simulink model "Powertrain_Simulation"  (R2017b)
settings: Solver=FixedStepAuto  StartTime=0.0  StopTime=Inf  MinStep=0.01  RelTol=1e-3
values from neighbouring files (symbols this model uses):
  Rear_Sprocket_FirstGear = Rear_Sprocket    [Optimize_SingleSpeedGearRatio.m]
  Rear_Sprocket_SecondGear = Rear_Sprocket    [Optimize_SingleSpeedGearRatio.m]
undefined symbols (not defined in the file or in its folder): A1, AIR, C1, C2, COOLANT, cp, Elevation_Profile, EM, flowrate, hA1, k12, M, M2, MOT, RAD, Velocity_Profile
libraries: simulink x5
(part 1 of 2)
settings Model: Creator=salyer.103  LastModifiedBy=ra067402
settings SolverCC: ZeroCrossAlgorithm=Adaptive
settings CodeAppCC: StateflowObjectComments=on

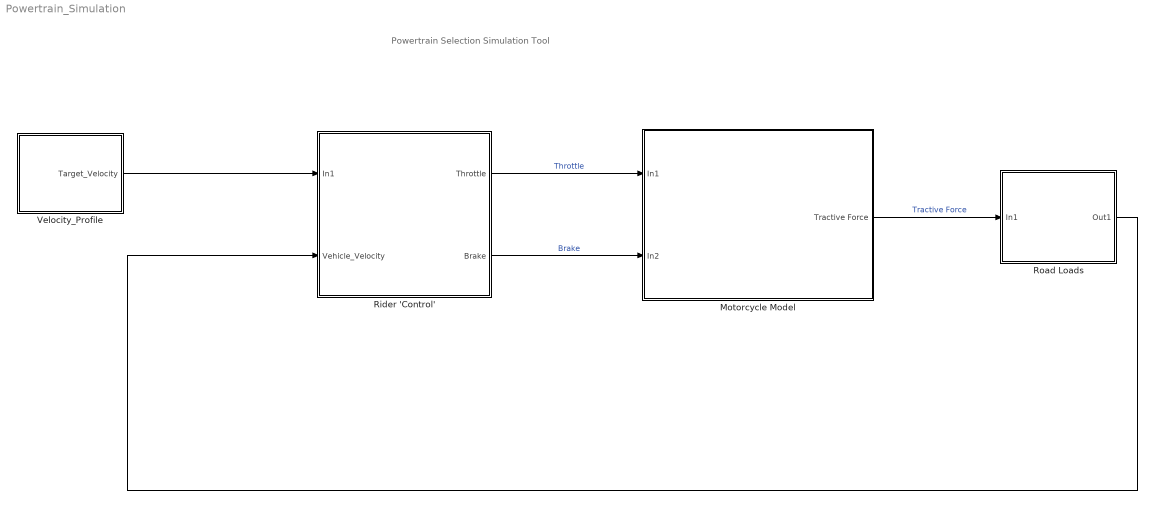
== system Powertrain_Simulation ==
  note: Powertrain Selection Simulation Tool
  Motorcycle Model : Subsystem  mask{Wheel_Radius=0.3, Final_Drive_Eff=0.92, Max_Brake_Torque=4000, Total_Mass=330, EM_MC_Selection=Ideal_TomegaCurve, b=0.728, h=0.72, g=9.81, p=1.4, mu_r=1, Front_Sprocket=21, Regen_Percent=100}
      mask prompts: Wheel_Radius "Wheel Radius (m)"; Final_Drive_Eff "Efficiency of Drivetrain"; Max_Brake_Torque "Maximum Braking Torque (Nm)"; Total_Mass "Vehicle Total Mass (kg)"; EM_MC_Selection "Motor-MC Combo"; b "Distance from Rear Wheel to CG (m)"; h "Height of CG from ground (m)"; g "Gravity (m/s2)"; p "Wheelbase (m)"; mu_r "Rear Wheel Coefficient of Friction"; Front_Sprocket "Front Sprocket Teeth"; Regen_Percent "Percentage of Max Regen (%)"
      mask init:
      | Initialize_Powertrain
      mask TypeOptions EM_MC_Selection: emrax268_pm150dz | RemyHVH25090s | Ideal_TomegaCurve
      mask Display: image('\\home2.coeit.osu.edu\s\salyer.103\Documents\GrabCAD\RW-4\Layout Space\Zach Salyer\Powertrain Simulation\Mask Pictures\bike.JPG');
  Rider 'Control' : Subsystem  mask{kp=5, ki=0, kd=0}
      mask Display: image('\\home2.coeit.osu.edu\s\salyer.103\Documents\GrabCAD\RW-4\Layout Space\Zach Salyer\Powertrain Simulation\Mask Pictures\helmet.jpg');
  Road Loads : Subsystem  mask{rowA=1, Wind_Speed=0, Cda=0.38, ElevationProfile=IOM_Elevation_Profile}
      mask prompts: rowA "Air Density"; Wind_Speed "Wind Speed (m/s)"; Cda "Cd * Frontal Area"; ElevationProfile "Course Elevation Profile"
      mask init:
      | Initialize_Elevation
      mask TypeOptions ElevationProfile: IOM_Elevation_Profile
  Velocity_Profile : Subsystem  mask{Circuit_Selection=IOM}
      mask prompts: Circuit_Selection "Circuit"
      mask init:
      | Initialize_Circuit
      mask TypeOptions Circuit_Selection: IOM
      mask Display: image('\\home2.coeit.osu.edu\s\salyer.103\Documents\GrabCAD\RW-4\Layout Space\Zach Salyer\Powertrain Simulation\Mask Pictures\VelocityProfile.png');
  wires:
  Velocity_Profile/1(Target_Velocity) -> Rider 'Control'/1(In1)
  Rider 'Control'/1(Throttle) -> Motorcycle Model/1(In1)  "Throttle"
  Rider 'Control'/2(Brake) -> Motorcycle Model/2(In2)  "Brake"
  Motorcycle Model/1(Tractive Force) -> Road Loads/1(In1)  "Tractive Force"
  Road Loads/1(Out1) -> Rider 'Control'/2(Vehicle_Velocity)

== system Powertrain_Simulation/Motorcycle Model ==
  note: When Rear Braking Strategy is added, will need to move pack energy req block
      | B/c negative torque applied gives regen to pack
      |
      | To determine actual applied torque prior to the wheel block we will  need to modulate torque based on
      | wheel slip from the rider model
  In1 : Inport
  In2 : Inport  Port=2
  Braking/Throttle Strategy : Subsystem
  Front Brakes : Subsystem
      mask Display: image('\\home2.coeit.osu.edu\s\salyer.103\Documents\GrabCAD\RW-4\Layout Space\Zach Salyer\Powertrain Simulation\Mask Pictures\motoBrake.JPG');
  Front Wheel (Limits Tractive Force) : Subsystem
      mask Display: image('\\home2.coeit.osu.edu\s\salyer.103\Documents\GrabCAD\RW-4\Layout Space\Zach Salyer\Powertrain Simulation\Mask Pictures\frTire_pirelli.JPG');
  Pack Energy Req : Subsystem
      mask Display: image('\\home2.coeit.osu.edu\s\salyer.103\Documents\GrabCAD\RW-4\Layout Space\Zach Salyer\Powertrain Simulation\Mask Pictures\pack.JPG');
  Powertrain : Subsystem
      mask Display: image('\\home2.coeit.osu.edu\s\salyer.103\Documents\GrabCAD\RW-4\Layout Space\Zach Salyer\Powertrain Simulation\Mask Pictures\bike_powertrain.JPG');
  Rear Brakes : Subsystem
      mask Display: image('\\home2.coeit.osu.edu\s\salyer.103\Documents\GrabCAD\RW-4\Layout Space\Zach Salyer\Powertrain Simulation\Mask Pictures\motoBrake.JPG');
  Rear Wheel (Limits Tractive Force) : Subsystem
      mask Display: image('\\home2.coeit.osu.edu\s\salyer.103\Documents\GrabCAD\RW-4\Layout Space\Zach Salyer\Powertrain Simulation\Mask Pictures\rrTire_pirelli.JPG');
  Sum : Sum  Inputs=+|+
  Sum1 : Sum  Inputs=++|
  To Workspace : ToWorkspace  VariableName=RearWhlForce  SampleTime=-1
  To Workspace1 : ToWorkspace  VariableName=FrontWhlForce  SaveFormat=Timeseries  SampleTime=-1
  Transmission : Subsystem
      mask Display: image('\\home2.coeit.osu.edu\s\salyer.103\Documents\GrabCAD\RW-4\Layout Space\Zach Salyer\Powertrain Simulation\Mask Pictures\gear.jpg');
  Vehicle Parameters : Subsystem
  Tractive Force : Outport
  wires:
  Sum/1 -> Tractive Force/1  "Tractive Force"
  Powertrain/1(Motor Torque) -> Transmission/1(Motor Torque)
  Front Brakes/1(Front Wheel Torque) -> Front Wheel (Limits Tractive Force)/1(In1)
  Front Wheel (Limits Tractive Force)/1(Out2) -> To Workspace1/1, Sum/2
  Rear Wheel (Limits Tractive Force)/1(Out1) -> To Workspace/1, Sum/1, Pack Energy Req/1(In1)
  In1/1 -> Braking/Throttle Strategy/1(In1)  "Throttle"
  Braking/Throttle Strategy/2(Out2) -> Powertrain/1(Throttle)
  In2/1 -> Braking/Throttle Strategy/2(In2)  "Brake"
  Braking/Throttle Strategy/3(Out3) -> Front Brakes/1(Throttle)
  Transmission/1(Out1) -> Sum1/2  "Motor Torque"
  Rear Brakes/1(Front Wheel Torque) -> Sum1/1  "Rear Brake Torque"
  Sum1/1 -> Rear Wheel (Limits Tractive Force)/1(In1)  "Total Torque"
  Braking/Throttle Strategy/1(Out1) -> Rear Brakes/1(Throttle)

== system Powertrain_Simulation/Rider 'Control' ==
  note: Note: This literally just does full throttle is speed < target speed and full brake if speed > target speed
      |
      | It also has a very small derivative gain to keep the simulation from getting stuck if speed = target speed
  note: If positive, accelerate
      | If negative, brake
  note: Tune PID Controller Later/Make Improved Rider Model
  In1 : Inport
  Vehicle_Velocity : Inport  Port=2
  " " : Gain  Gain=ki
  "  " : Gain  Gain=kp
  "   " : Gain  Gain=kd
  Brake Limit : Saturate  UpperLimit=0  LowerLimit=-1  ZeroCross=off
  Derivative : Derivative
  Integrator : Integrator
  Make Brake 0 or 1 : Rounding
  Make Throttle 0 or 1 : Rounding  Operator=ceil
  Scope : Scope
  Sum : Sum  Inputs=+-
  Sum1 : Sum  Inputs=+++
  T : Scope
  Throttle Limit : Saturate  UpperLimit=1  LowerLimit=0  ZeroCross=off
  Throttle : Outport
  Brake : Outport  Port=2
  wires:
  Vehicle_Velocity/1 -> Sum/2  "Velocity"
  In1/1 -> Scope/1, Sum/1  "Target_Velocity"
  "  "/1 -> Sum1/1
  Sum/1 -> "  "/1, " "/1, "   "/1
  Throttle Limit/1 -> Make Throttle 0 or 1/1  "Throttle"
  Make Throttle 0 or 1/1 -> T/1, Throttle/1
  Make Brake 0 or 1/1 -> Brake/1
  " "/1 -> Integrator/1
  Integrator/1 -> Sum1/2
  "   "/1 -> Derivative/1
  Derivative/1 -> Sum1/3
  Sum1/1 -> Brake Limit/1, Throttle Limit/1
  Brake Limit/1 -> Make Brake 0 or 1/1  "Brake"

== system Powertrain_Simulation/Road Loads ==
  In1 : Inport
  Enviornment : Subsystem
  To Workspace : ToWorkspace  VariableName=Vehicle_Velocity  SampleTime=-1
      settings: Save2DSignal=2-D array (concatenate along first dimension)
  To Workspace1 : ToWorkspace  VariableName=resistanceforce  SampleTime=-1
      settings: Save2DSignal=2-D array (concatenate along first dimension)
  Vehicle Loads : Subsystem
  Vehicle_speed_Calculation : Subsystem
  Out1 : Outport
  tag scope: Vehicle_Velocity_ms=global
  wires:
  In1/1 -> Vehicle_speed_Calculation/1(In1)  "Tractive Force"
  Vehicle_speed_Calculation/1(F (N)1) -> To Workspace/1, Out1/1, [Vehicle_Velocity_ms]  "Velocity"
  Vehicle Loads/1(F (N)) -> To Workspace1/1, Vehicle_speed_Calculation/2(In3)

== system Powertrain_Simulation/Velocity_Profile ==
  Constant : Constant  Value=Velocity_Profile.distance(end)
  Relational Operator1 : RelationalOperator  RndMeth=Nearest  InputSameDT=on
  Stop Simulation : Stop
  Vehicle_Target_Speed : Lookup  InputValues=Velocity_Profile.distance  Table=Velocity_Profile.velocity  LookUpMeth=Interpolation-Use End Values  SaturateOnIntegerOverflow=on
  Target_Velocity : Outport
  wires:
  Vehicle_Target_Speed/1 -> Target_Velocity/1  "Target_Velocity"
  Constant/1 -> Relational Operator1/2
  Relational Operator1/1 -> Stop Simulation/1
  [Distance_Total_m] -> Relational Operator1/1, Vehicle_Target_Speed/1

== system Powertrain_Simulation/Motorcycle Model/Braking//Throttle Strategy ==
  note: Notes:
      | -No Rear Brake currently being used, no point in using it until we have a better rider model
      | -If throttle = 0, then switch to -1 to request negative torque
      | -All brake request is front brake
  In1 : Inport
  In2 : Inport  Port=2
  Constant : Constant  Value=0
  Constant1 : Constant  Value=-1
  Gain : Gain
  Switch : Switch  Criteria=u2 > Threshold
  Out1 : Outport
  Out2 : Outport  Port=2
  Out3 : Outport  Port=3
  wires:
  Constant/1 -> Out1/1  "Rear Brake Request"
  In1/1 -> Switch/1, Switch/2  "Throttle Request"
  In2/1 -> Gain/1  "Brake Request"
  Gain/1 -> Out3/1  "Front Brake Request"
  Constant1/1 -> Switch/3
  Switch/1 -> Out2/1  "Torque Request"

== system Powertrain_Simulation/Motorcycle Model/Front Brakes ==
  Throttle : Inport
  Multiply : Product  Inputs=**
  Front Wheel Torque : Outport
  wires:
  Throttle/1 -> Multiply/1  "Brake"
  [Max_Brake_Torque] -> Multiply/2
  Multiply/1 -> Front Wheel Torque/1  "Front Wheel Torque"

== system Powertrain_Simulation/Motorcycle Model/Front Wheel (Limits Tractive Force) ==
  In1 : Inport
  Constant : Constant  Value=0
  Constant1 : Constant  Value=0
  Divide : Product  Inputs=*/
  Dynamic Front Wheel Load * mu : Fcn  Expr=-mu_r*Total_Mass*g*b/p + u(1)*h/p
  Stoppie Limit Brake Force : Constant  Value=-Total_Mass*g*(p-b)/h
  Stoppie Limited Brake Force : simulink/Discontinuities/Saturation Dynamic  OutMin=[]  OutMax=[]  OutDataTypeStr=Inherit: Same as second input  OutDataType=fixdt(1, 16)  OutScaling=2^-10  DoSatur=off
  Sum1 : Sum
  To Workspace : ToWorkspace  VariableName=FrictionLimit  SaveFormat=Timeseries  SampleTime=-1
  Traction Limited Brake Force : simulink/Discontinuities/Saturation Dynamic  OutMin=[]  OutMax=[]  OutDataTypeStr=Inherit: Same as second input  OutDataType=fixdt(1, 16)  OutScaling=2^-10  DoSatur=off
  Out2 : Outport
  tag scope: Front_Brake_Force=global
  wires:
  In1/1 -> Divide/1  "Front Wheel Torque"
  Stoppie Limited Brake Force/1 -> [Front_Brake_Force], Out2/1  "Tractive Force"
  Divide/1 -> Traction Limited Brake Force/2
  [Fr_Wheel_Radius] -> Divide/2
  [Front_Brake_Force] -> Sum1/1
  [Rear_Brake_Force] -> Sum1/2
  Sum1/1 -> Dynamic Front Wheel Load * mu/1
  Dynamic Front Wheel Load * mu/1 -> To Workspace/1, Traction Limited Brake Force/3
  Constant/1 -> Traction Limited Brake Force/1
  Traction Limited Brake Force/1 -> Stoppie Limited Brake Force/2
  Constant1/1 -> Stoppie Limited Brake Force/1
  Stoppie Limit Brake Force/1 -> Stoppie Limited Brake Force/3

== system Powertrain_Simulation/Motorcycle Model/Pack Energy Req ==
  In1 : Inport
  Convert W-s to kW-h : Gain  Gain=1/3600/1000
  Divide : Product  Inputs=*/
  Gain : Gain  Gain=1/1000
  Integrator : Integrator
  Product : Product
  Product1 : Product
  To Workspace : ToWorkspace  VariableName=Motor_Torque_Limited  SampleTime=-1
      settings: Save2DSignal=2-D array (concatenate along first dimension)
  To Workspace1 : ToWorkspace  VariableName=Power  SampleTime=-1
      settings: Save2DSignal=2-D array (concatenate along first dimension)
  To Workspace2 : ToWorkspace  VariableName=Energy_req  SampleTime=-1
      settings: Save2DSignal=2-D array (concatenate along first dimension)
  rpm to rad/s : Gain  Gain=1/60*2*pi
  wires:
  In1/1 -> Product1/1  "Tractive Force"
  Convert W-s to kW-h/1 -> To Workspace2/1
  [EM_RPM] -> rpm to rad/s/1
  Integrator/1 -> Convert W-s to kW-h/1  "Energy"
  rpm to rad/s/1 -> Product/2
  Product/1 -> Gain/1, Integrator/1  "Power (W)"
  Divide/1 -> To Workspace/1, Product/1  "Motor Torque Actual"
  [Rr_Wheel_Radius] -> Product1/2
  Product1/1 -> Divide/1  "Whl Torque"
  [Final_Drive_Ratio] -> Divide/2
  Gain/1 -> To Workspace1/1

== system Powertrain_Simulation/Motorcycle Model/Powertrain ==
  note: Find max torque available based on RPM
  note: Apply max torque (sign will depend on if throttle is positive or negative - regen or accelerate)
      | Apply gain for regen percentage to decrease from max torque is desired
  Throttle : Inport
  Divide : Product  Inputs=**
  EM Max Torque Curve : Lookup  InputValues=EM.N_RPM  Table=EM.T_max_Peak  LookUpMeth=Interpolation-Use End Values  SaturateOnIntegerOverflow=on
  Gain : Gain  Gain=Regen_Percent/100
  Goto : Goto  Commented=on  GotoTag=EM_Torque  TagVisibility=global
  Powertrain Thermal Model : Subsystem  Commented=on
  Switch : Switch  Criteria=u2 > Threshold
  To Workspace : ToWorkspace  VariableName=EM_RPM  SampleTime=-1
      settings: Save2DSignal=2-D array (concatenate along first dimension)
  To Workspace2 : ToWorkspace  VariableName=motorT  SaveFormat=Timeseries  SampleTime=-1
  Motor Torque : Outport
  wires:
  Throttle/1 -> Divide/1  "Throttle"
  Divide/1 -> To Workspace2/1, Goto/1, Switch/2, Gain/1, Switch/1  "Motor Torque"
  [EM_RPM] -> To Workspace/1, EM Max Torque Curve/1  "EM_RPM"
  EM Max Torque Curve/1 -> [T_Max_from_EM]  "Max Torque"
  [T_Max_from_EM] -> Divide/2
  Switch/1 -> Motor Torque/1  "Motor Torque"
  Gain/1 -> Switch/3

== system Powertrain_Simulation/Motorcycle Model/Rear Brakes ==
  Throttle : Inport
  Multiply : Product  Inputs=**
  Front Wheel Torque : Outport
  wires:
  Throttle/1 -> Multiply/1  "Brake"
  [Max_Brake_Torque] -> Multiply/2
  Multiply/1 -> Front Wheel Torque/1  "Rear Wheel Torque"

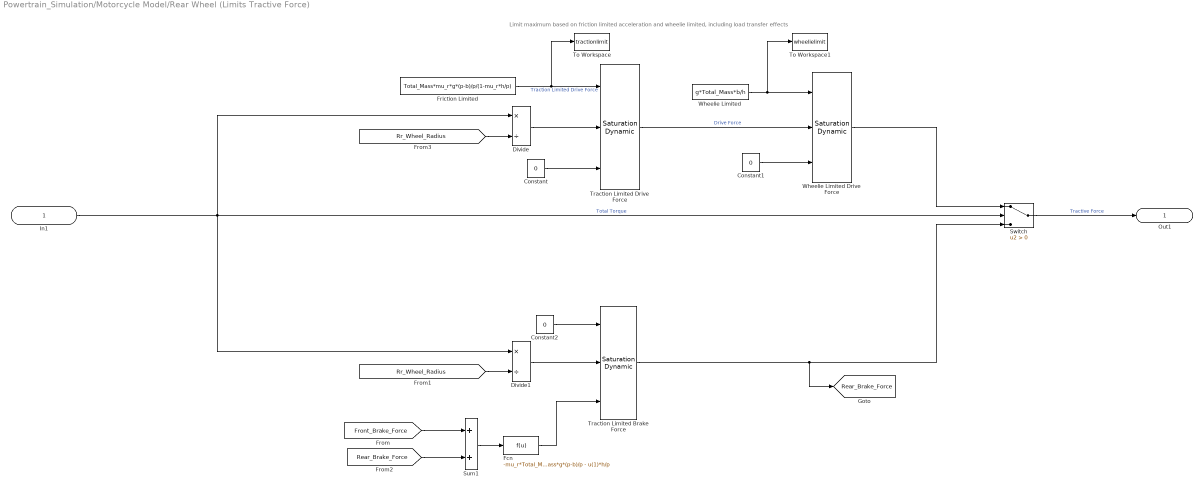
== system Powertrain_Simulation/Motorcycle Model/Rear Wheel (Limits Tractive Force) ==
  note: Limit maximum based on friction limited acceleration and wheelie limited, including load transfer effects
  In1 : Inport
  Constant : Constant  Value=0
  Constant1 : Constant  Value=0
  Constant2 : Constant  Value=0
  Divide : Product  Inputs=*/
  Divide1 : Product  Inputs=*/
  Fcn : Fcn  Expr=-mu_r*Total_Mass*g*(p-b)/p - u(1)*h/p
  Friction Limited : Constant  Value=Total_Mass*mu_r*g*(p-b)/p/(1-mu_r*h/p)
  Sum1 : Sum
  Switch : Switch  Criteria=u2 > Threshold
  To Workspace : ToWorkspace  VariableName=tractionlimit  SaveFormat=Timeseries  SampleTime=-1
  To Workspace1 : ToWorkspace  VariableName=wheelielimit  SaveFormat=Timeseries  SampleTime=-1
  Traction Limited Brake Force : simulink/Discontinuities/Saturation Dynamic  OutMin=[]  OutMax=[]  OutDataTypeStr=Inherit: Same as second input  OutDataType=fixdt(1, 16)  OutScaling=2^-10  DoSatur=off
  Traction Limited Drive Force : simulink/Discontinuities/Saturation Dynamic  OutMin=[]  OutMax=[]  OutDataTypeStr=Inherit: Same as second input  OutDataType=fixdt(1, 16)  OutScaling=2^-10  DoSatur=off
  Wheelie Limited : Constant  Value=g*Total_Mass*b/h
  Wheelie Limited Drive Force : simulink/Discontinuities/Saturation Dynamic  OutMin=[]  OutMax=[]  OutDataTypeStr=Inherit: Same as second input  OutDataType=fixdt(1, 16)  OutScaling=2^-10  DoSatur=off
  Out1 : Outport
  tag scope: Rear_Brake_Force=global
  wires:
  [Rr_Wheel_Radius] -> Divide/2
  Friction Limited/1 -> To Workspace/1, Traction Limited Drive Force/1  "Traction Limited Drive Force"
  Traction Limited Drive Force/1 -> Wheelie Limited Drive Force/2  "Drive Force"
  Constant/1 -> Traction Limited Drive Force/3
  Constant1/1 -> Wheelie Limited Drive Force/3
  Wheelie Limited/1 -> To Workspace1/1, Wheelie Limited Drive Force/1
  Divide/1 -> Traction Limited Drive Force/2
  In1/1 -> Divide/1, Switch/2, Divide1/1  "Total Torque"
  [Rr_Wheel_Radius] -> Divide1/2
  Divide1/1 -> Traction Limited Brake Force/2
  Switch/1 -> Out1/1  "Tractive Force"
  Wheelie Limited Drive Force/1 -> Switch/1
  Traction Limited Brake Force/1 -> Switch/3, [Rear_Brake_Force]
  Constant2/1 -> Traction Limited Brake Force/1
  [Front_Brake_Force] -> Sum1/1
  [Rear_Brake_Force] -> Sum1/2
  Sum1/1 -> Fcn/1
  Fcn/1 -> Traction Limited Brake Force/3

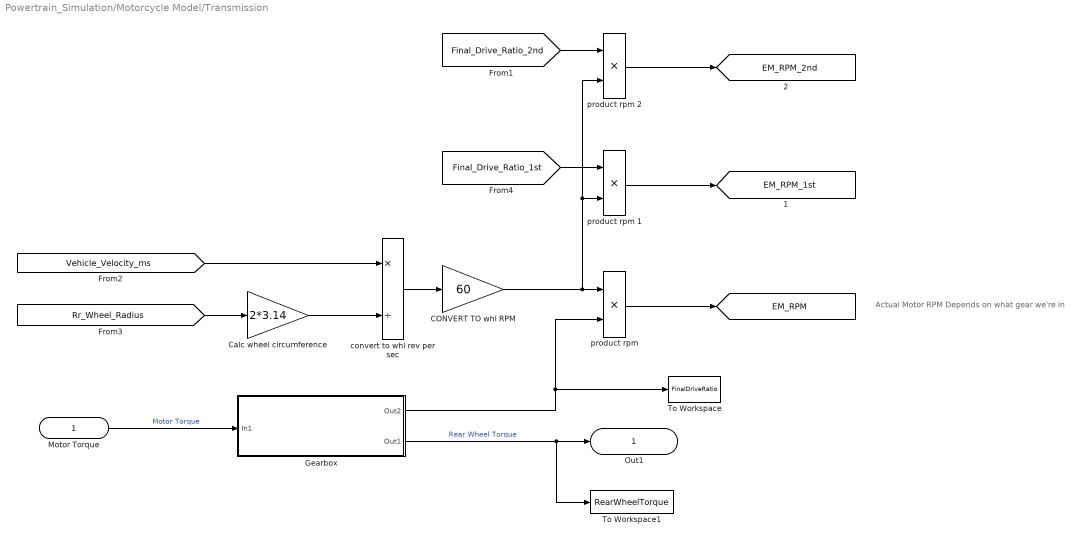
== system Powertrain_Simulation/Motorcycle Model/Transmission ==
  note: Actual Motor RPM Depends on what gear we're in
  Motor Torque : Inport
  "CONVERT TO whl RPM " : Gain  Gain=60
  Calc wheel circumference : Gain  Gain=2*3.14
  "Gearbox " : Subsystem
  To Workspace : ToWorkspace  VariableName=FinalDriveRatio  SampleTime=-1
      settings: Save2DSignal=2-D array (concatenate along first dimension)
  To Workspace1 : ToWorkspace  VariableName=RearWheelTorque  SampleTime=-1
      settings: Save2DSignal=2-D array (concatenate along first dimension)
  "convert to whl rev per sec " : Product  Inputs=*/
  "product rpm " : Product  Inputs=**
  product rpm 1 : Product  Inputs=**
  product rpm 2 : Product  Inputs=**
  Out1 : Outport
  tag scope: EM_RPM=global, EM_RPM_1st=global, EM_RPM_2nd=global
  wires:
  "Gearbox "/2(Out1) -> To Workspace1/1, Out1/1  "Rear Wheel Torque"
  Calc wheel circumference/1 -> "convert to whl rev per sec "/2
  [Vehicle_Velocity_ms] -> "convert to whl rev per sec "/1
  [Rr_Wheel_Radius] -> Calc wheel circumference/1
  "convert to whl rev per sec "/1 -> "CONVERT TO whl RPM "/1
  "product rpm "/1 -> [EM_RPM]
  Motor Torque/1 -> "Gearbox "/1(In1)  "Motor Torque"
  "CONVERT TO whl RPM "/1 -> product rpm 2/2, product rpm 1/2, "product rpm "/1
  [Final_Drive_Ratio_1st] -> product rpm 1/1
  [Final_Drive_Ratio_2nd] -> product rpm 2/1
  product rpm 1/1 -> [EM_RPM_1st]
  product rpm 2/1 -> [EM_RPM_2nd]
  "Gearbox "/1(Out2) -> To Workspace/1, "product rpm "/2

== system Powertrain_Simulation/Motorcycle Model/Vehicle Parameters ==
  Constant : Constant  Value=Total_Mass
  Divide : Product  Inputs=*/
  Divide1 : Product  Inputs=*/
  Final_Drive_Eff : Constant  Value=Final_Drive_Eff
  Front_Sprocket_Teeth : Constant  Value=Front_Sprocket
  Front_Sprocket_Teeth1 : Constant  Value=Front_Sprocket
  Max_Brake_Torque : Constant  Value=Max_Brake_Torque
  Rear_Sprocket_Teeth : Constant  Value=Rear_Sprocket_FirstGear
  Rear_Sprocket_Teeth1 : Constant  Value=Rear_Sprocket_SecondGear
  Wheel_Radius : Constant  Value=Wheel_Radius
  tag scope: Final_Drive_Eff=global, Final_Drive_Ratio_1st=global, Final_Drive_Ratio_2nd=global, Fr_Wheel_Radius=global, Mass=global, Max_Brake_Torque=global, Rr_Wheel_Radius=global
  wires:
  Wheel_Radius/1 -> [Rr_Wheel_Radius], [Fr_Wheel_Radius]
  Front_Sprocket_Teeth/1 -> Divide/2
  Rear_Sprocket_Teeth/1 -> Divide/1
  Final_Drive_Eff/1 -> [Final_Drive_Eff]
  Max_Brake_Torque/1 -> [Max_Brake_Torque]
  Constant/1 -> [Mass]
  Divide/1 -> [Final_Drive_Ratio_1st]
  Divide1/1 -> [Final_Drive_Ratio_2nd]
  Rear_Sprocket_Teeth1/1 -> Divide1/1
  Front_Sprocket_Teeth1/1 -> Divide1/2

== system Powertrain_Simulation/Road Loads/Enviornment ==
  Constant : Constant  Value=Cda
  Constant1 : Constant  Value=Wind_Speed
  Constant4 : Constant  Value=rowA
  tag scope: Cda=global, Row_Air=global, Wind_Speed=global
  wires:
  Constant1/1 -> [Wind_Speed]  "wind speed"
  Constant4/1 -> [Row_Air]  "air density"
  Constant/1 -> [Cda]

== system Powertrain_Simulation/Road Loads/Vehicle Loads ==
  Aerodynamic  Drag : Subsystem
  Grade Force : Subsystem
  Roll Force : Subsystem
  Sum4 : Sum  Inputs=+++
  To Workspace : ToWorkspace  VariableName=gradeforce  SampleTime=-1
  F (N) : Outport
  wires:
  Sum4/1 -> F (N)/1  "Road Load (N)"
  Roll Force/1(Power_roll) -> Sum4/3
  Aerodynamic  Drag/1(Drag Power) -> Sum4/2
  Grade Force/1(Drag Power) -> To Workspace/1, Sum4/1  "Grade Force"

== system Powertrain_Simulation/Road Loads/Vehicle_speed_Calculation ==
  In1 : Inport
  In3 : Inport  Port=2
  Divide : Product  Inputs=*/
  Integrator Limited : Integrator  LimitOutput=on  LowerSaturationLimit=0
  Integrator Limited1 : Integrator  LimitOutput=on  LowerSaturationLimit=0
  Sum : Sum  Inputs=+-
  To Workspace : ToWorkspace  VariableName=Vehicle_Distance  SampleTime=-1
      settings: Save2DSignal=2-D array (concatenate along first dimension)
  F (N)1 : Outport
  tag scope: Distance_Total_m=global
  wires:
  Sum/1 -> Divide/1  "Net_Force"
  Divide/1 -> Integrator Limited/1  "Vehicle_Acceleration"
  In1/1 -> Sum/1
  [Mass] -> Divide/2
  In3/1 -> Sum/2
  Integrator Limited/1 -> F (N)1/1, Integrator Limited1/1  "vehicle_speed"
  Integrator Limited1/1 -> To Workspace/1, [Distance_Total_m]  "distance"

== system Powertrain_Simulation/Motorcycle Model/Powertrain/Powertrain Thermal Model ==
  Constant : Constant
  EMRAX Motor Thermal Model : Subsystem
  Radiator Thermal Model : Subsystem
  Reinhardt Inverter Thermal Model : Subsystem
  To Workspace1 : ToWorkspace  VariableName=Stator_Temp  SaveFormat=Timeseries  SampleTime=-1
  To Workspace3 : ToWorkspace  VariableName=Rotor_Temp  SaveFormat=Timeseries  SampleTime=-1
  To Workspace4 : ToWorkspace  VariableName=Motor_Mounting_Temp  SaveFormat=Timeseries  SampleTime=-1
  wires:
  [EM_RPM] -> EMRAX Motor Thermal Model/1(Motor Speed [rpm])
  [EM_Torque] -> EMRAX Motor Thermal Model/2(Motor Torque [Nm])
  Constant/1 -> EMRAX Motor Thermal Model/3(Motor ON Flag [-])
  EMRAX Motor Thermal Model/2(T_mass_2 [K]) -> To Workspace3/1
  EMRAX Motor Thermal Model/1(T_mass_1 [K]) -> To Workspace1/1
  EMRAX Motor Thermal Model/4(T_mass_3 [K]1) -> To Workspace4/1
  [Pack_Voltage] -> Reinhardt Inverter Thermal Model/1(In1)
  [Inverter_Cool_in] -> Reinhardt Inverter Thermal Model/3(In3)
  [Motor_Cool_in] -> EMRAX Motor Thermal Model/4(Temp_cool_RAD_out [K])

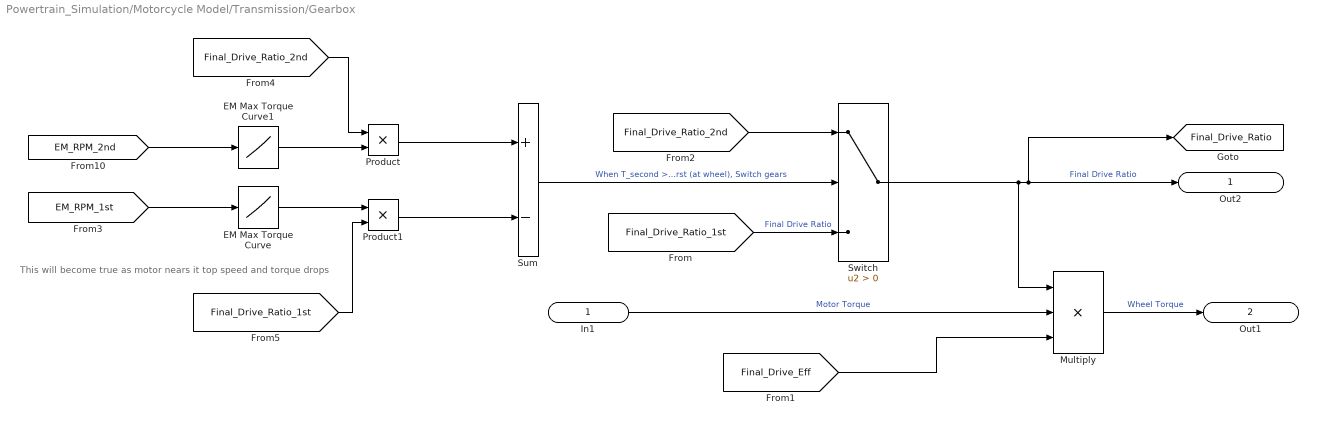
== system Powertrain_Simulation/Motorcycle Model/Transmission/Gearbox  ==
  note: This will become true as motor nears it top speed and torque drops
  In1 : Inport
  EM Max Torque Curve : Lookup  InputValues=EM.N_RPM  Table=EM.T_max_Peak  LookUpMeth=Interpolation-Use End Values  SaturateOnIntegerOverflow=on
  EM Max Torque Curve1 : Lookup  InputValues=EM.N_RPM  Table=EM.T_max_Peak  LookUpMeth=Interpolation-Use End Values  SaturateOnIntegerOverflow=on
  Multiply : Product  Inputs=***
  Product : Product
  Product1 : Product
  Sum : Sum  Inputs=+-
  Switch : Switch  Criteria=u2 > Threshold
  Out2 : Outport
  Out1 : Outport  Port=2
  tag scope: Final_Drive_Ratio=global
  wires:
  [Final_Drive_Eff] -> Multiply/3
  Multiply/1 -> Out1/1  "Wheel Torque"
  In1/1 -> Multiply/2  "Motor Torque"
  [Final_Drive_Ratio_1st] -> Switch/3  "Final Drive Ratio"
  [Final_Drive_Ratio_2nd] -> Switch/1
  Sum/1 -> Switch/2  "When T_second > T_First (at wheel), Switch gears"
  Switch/1 -> [Final_Drive_Ratio], Out2/1, Multiply/1  "Final Drive Ratio"
  [EM_RPM_2nd] -> EM Max Torque Curve1/1
  [EM_RPM_1st] -> EM Max Torque Curve/1
  EM Max Torque Curve1/1 -> Product/2
  [Final_Drive_Ratio_2nd] -> Product/1
  EM Max Torque Curve/1 -> Product1/1
  [Final_Drive_Ratio_1st] -> Product1/2
  Product1/1 -> Sum/2
  Product/1 -> Sum/1

== system Powertrain_Simulation/Road Loads/Vehicle Loads/Aerodynamic  Drag ==
  Constant : Constant  Value=0.5
  Drag force =1/2*row_a*Cd*Af*v2 : Product  Inputs=4  RndMeth=Zero
  Sum : Sum  Inputs=|++
  drag_v1 : Math  Operator=pow  SaturateOnIntegerOverflow=on
  square : Constant  Value=2
  Drag Power : Outport
  wires:
  square/1 -> drag_v1/2
  Constant/1 -> Drag force =1/2*row_a*Cd*Af*v2/1
  [Cda] -> Drag force =1/2*row_a*Cd*Af*v2/3
  [Row_Air] -> Drag force =1/2*row_a*Cd*Af*v2/2
  Drag force =1/2*row_a*Cd*Af*v2/1 -> Drag Power/1  "Drag_Force (N)"
  [Vehicle_Velocity_ms] -> Sum/1
  Sum/1 -> drag_v1/1
  [Wind_Speed] -> Sum/2
  drag_v1/1 -> Drag force =1/2*row_a*Cd*Af*v2/4

== system Powertrain_Simulation/Road Loads/Vehicle Loads/Grade Force ==
  note: If grade force is NaN, apply 0 force, otherwise export grade force
  Constant : Constant  Value=0
  Divide : Product  Inputs=*/
  Elevation : Lookup  InputValues=Elevation_Profile.distance  Table=Elevation_Profile.elevation  LookUpMeth=Interpolation-Use End Values  SaturateOnIntegerOverflow=on
  Fcn : Fcn  Expr=sin(u)
  Fcn1 : Fcn  Expr=atan(u(1))
  Grade Force = M*g*sin(road_grade) : Product  Inputs=3  RndMeth=Zero
  Memory : Memory
  Past Elevation : Lookup  InputValues=Elevation_Profile.distance  Table=Elevation_Profile.elevation  LookUpMeth=Interpolation-Use End Values  SaturateOnIntegerOverflow=on
  Relational Operator : RelationalOperator  Operator=isNaN  OutDataTypeStr=boolean  RndMeth=Simplest
  Sum : Sum  Inputs=+-
  Sum1 : Sum  Inputs=-+
  Switch : Switch  Threshold=1
  gravity : Constant  Value=9.81
  Drag Power : Outport
  wires:
  Fcn1/1 -> Fcn/1
  [Mass] -> Grade Force = M*g*sin(road_grade)/1
  gravity/1 -> Grade Force = M*g*sin(road_grade)/2
  Divide/1 -> Fcn1/1
  Past Elevation/1 -> Sum/2
  Memory/1 -> Sum1/1, Past Elevation/1
  Sum/1 -> Divide/1  "Elevation change"
  Elevation/1 -> Sum/1
  [Distance_Total_m] -> Sum1/2, Memory/1, Elevation/1
  Sum1/1 -> Divide/2  "Distance Change"
  Fcn/1 -> Grade Force = M*g*sin(road_grade)/3
  Switch/1 -> Drag Power/1  "Grade_Force (N)"
  Grade Force = M*g*sin(road_grade)/1 -> Switch/3, Relational Operator/1  "Grade_Force(N)"
  Relational Operator/1 -> Switch/2
  Constant/1 -> Switch/1

== system Powertrain_Simulation/Road Loads/Vehicle Loads/Roll Force ==
  note: Create a more accurate estimate later (Cossalter has formulas)
  Aprrox. Rolling Resistance Force : Constant  Value=0.02
  Gravity (m/s2) : Constant  Value=9.81
  Product : Product  Inputs=3
  Power_roll : Outport
  wires:
  Product/1 -> Power_roll/1  "Roll_Force (N)"
  [Mass] -> Product/1
  Gravity (m/s2)/1 -> Product/2
  Aprrox. Rolling Resistance Force/1 -> Product/3

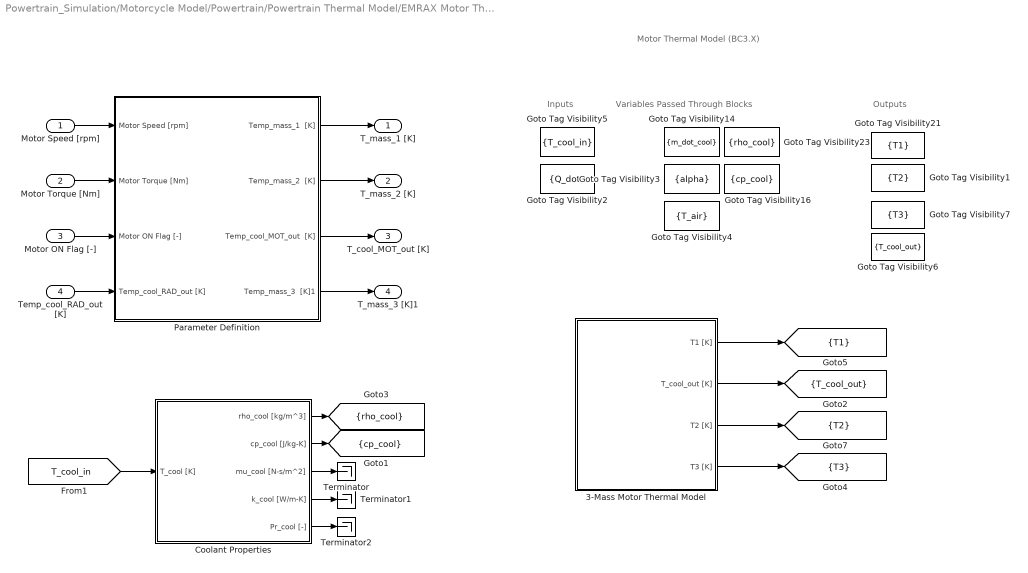
== system Powertrain_Simulation/Motorcycle Model/Powertrain/Powertrain Thermal Model/EMRAX Motor Thermal Model ==
  note: Variables Passed Through Blocks
  note: Inputs
  note: Motor Thermal Model
      | (BC3.X)
  note: Outputs
  Motor Speed [rpm] : Inport
  Motor Torque [Nm] : Inport  Port=2
  Motor ON Flag [-] : Inport  Port=3
  Temp_cool_RAD_out [K] : Inport  Port=4
  3-Mass Motor Thermal Model : Subsystem
  Coolant Properties : Subsystem
  Goto Tag Visibility1 : GotoTagVisibility  GotoTag=T2
  Goto Tag Visibility14 : GotoTagVisibility  GotoTag=m_dot_cool
  Goto Tag Visibility16 : GotoTagVisibility  GotoTag=cp_cool
  Goto Tag Visibility2 : GotoTagVisibility  GotoTag=Q_dot
  Goto Tag Visibility21 : GotoTagVisibility  GotoTag=T1
  Goto Tag Visibility23 : GotoTagVisibility  GotoTag=rho_cool
  Goto Tag Visibility3 : GotoTagVisibility  GotoTag=alpha
  Goto Tag Visibility4 : GotoTagVisibility  GotoTag=T_air
  Goto Tag Visibility5 : GotoTagVisibility  GotoTag=T_cool_in
  Goto Tag Visibility6 : GotoTagVisibility  GotoTag=T_cool_out
  Goto Tag Visibility7 : GotoTagVisibility  GotoTag=T3
  Parameter Definition : Subsystem
  Terminator : Terminator
  Terminator1 : Terminator
  Terminator2 : Terminator
  T_mass_1 [K] : Outport
  T_mass_2 [K] : Outport  Port=2
  T_cool_MOT_out [K] : Outport  Port=3
  T_mass_3 [K]1 : Outport  Port=4
  tag scope: T1=scoped, T2=scoped, T3=scoped, T_cool_out=scoped, cp_cool=scoped, rho_cool=scoped
  wires:
  Coolant Properties/1(rho_cool [kg/m^3]) -> [rho_cool]
  Coolant Properties/2(cp_cool [J/kg-K]) -> [cp_cool]
  [T_cool_in] -> Coolant Properties/1(T_cool [K])
  Coolant Properties/3(mu_cool [N-s/m^2]) -> Terminator/1
  Coolant Properties/4(k_cool [W/m-K]) -> Terminator1/1
  Coolant Properties/5(Pr_cool [-]) -> Terminator2/1
  3-Mass Motor Thermal Model/1(T1 [K]) -> [T1]
  3-Mass Motor Thermal Model/3(T2 [K]) -> [T2]
  Motor Torque [Nm]/1 -> Parameter Definition/2(Motor Torque [Nm])
  Motor ON Flag [-]/1 -> Parameter Definition/3(Motor ON Flag [-])
  Temp_cool_RAD_out [K]/1 -> Parameter Definition/4(Temp_cool_RAD_out [K])
  Parameter Definition/2(Temp_mass_2  [K]) -> T_mass_2 [K]/1
  Motor Speed [rpm]/1 -> Parameter Definition/1(Motor Speed [rpm])
  3-Mass Motor Thermal Model/2(T_cool_out [K]) -> [T_cool_out]
  Parameter Definition/3(Temp_cool_MOT_out  [K]) -> T_cool_MOT_out [K]/1
  Parameter Definition/1(Temp_mass_1  [K]) -> T_mass_1 [K]/1
  Parameter Definition/4(Temp_mass_3  [K]1) -> T_mass_3 [K]1/1
  3-Mass Motor Thermal Model/4(T3 [K]) -> [T3]

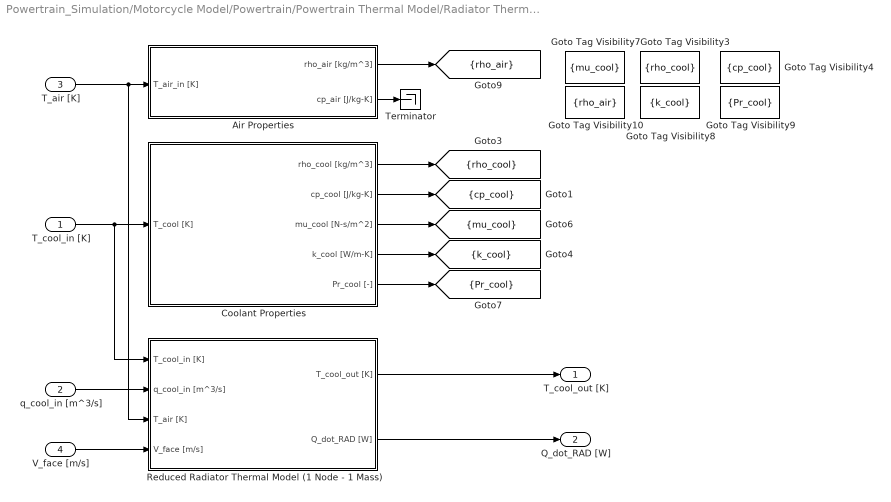
== system Powertrain_Simulation/Motorcycle Model/Powertrain/Powertrain Thermal Model/Radiator Thermal Model ==
  T_cool_in [K] : Inport
  q_cool_in [m^3/s] : Inport  Port=2
  T_air [K] : Inport  Port=3
  V_face [m/s] : Inport  Port=4
  Air Properties : Subsystem
  Coolant Properties : Subsystem
  Goto Tag Visibility10 : GotoTagVisibility  GotoTag=rho_air
  Goto Tag Visibility3 : GotoTagVisibility  GotoTag=rho_cool
  Goto Tag Visibility4 : GotoTagVisibility  GotoTag=cp_cool
  Goto Tag Visibility7 : GotoTagVisibility  GotoTag=mu_cool
  Goto Tag Visibility8 : GotoTagVisibility  GotoTag=k_cool
  Goto Tag Visibility9 : GotoTagVisibility  GotoTag=Pr_cool
  Reduced Radiator Thermal Model (1 Node - 1 Mass) : Subsystem
  Terminator : Terminator
  T_cool_out [K] : Outport
  Q_dot_RAD [W] : Outport  Port=2
  tag scope: Pr_cool=scoped, cp_cool=scoped, k_cool=scoped, mu_cool=scoped, rho_air=scoped, rho_cool=scoped
  wires:
  Coolant Properties/4(k_cool [W/m-K]) -> [k_cool]
  Air Properties/1(rho_air [kg/m^3]) -> [rho_air]
  Reduced Radiator Thermal Model (1 Node - 1 Mass)/2(Q_dot_RAD [W]) -> Q_dot_RAD [W]/1
  Coolant Properties/2(cp_cool [J/kg-K]) -> [cp_cool]
  T_air [K]/1 -> Reduced Radiator Thermal Model (1 Node - 1 Mass)/3(T_air [K]), Air Properties/1(T_air_in [K])
  Reduced Radiator Thermal Model (1 Node - 1 Mass)/1(T_cool_out [K]) -> T_cool_out [K]/1
  T_cool_in [K]/1 -> Reduced Radiator Thermal Model (1 Node - 1 Mass)/1(T_cool_in [K]), Coolant Properties/1(T_cool [K])
  Air Properties/2(cp_air [J/kg-K]) -> Terminator/1
  q_cool_in [m^3/s]/1 -> Reduced Radiator Thermal Model (1 Node - 1 Mass)/2(q_cool_in [m^3/s])
  V_face [m/s]/1 -> Reduced Radiator Thermal Model (1 Node - 1 Mass)/4(V_face [m/s])
  Coolant Properties/5(Pr_cool [-]) -> [Pr_cool]
  Coolant Properties/1(rho_cool [kg/m^3]) -> [rho_cool]
  Coolant Properties/3(mu_cool [N-s/m^2]) -> [mu_cool]

== system Powertrain_Simulation/Motorcycle Model/Powertrain/Powertrain Thermal Model/Reinhardt Inverter Thermal Model ==
  In1 : Inport
  In2 : Inport  Port=2
  In3 : Inport  Port=3
  Coolant Properties : Subsystem
  Inverter Thermal Model : Subsystem
  Terminator : Terminator
  Terminator1 : Terminator
  Terminator2 : Terminator
  Out1 : Outport
  Out2 : Outport  Port=2
  Out3 : Outport  Port=3
  tag scope: cp_cool=scoped, rho_cool=scoped
  wires:
  Coolant Properties/3(mu_cool [N-s/m^2]) -> Terminator/1
  Coolant Properties/5(Pr_cool [-]) -> Terminator2/1
  Coolant Properties/1(rho_cool [kg/m^3]) -> [rho_cool]
  Coolant Properties/4(k_cool [W/m-K]) -> Terminator1/1
  Coolant Properties/2(cp_cool [J/kg-K]) -> [cp_cool]
  Inverter Thermal Model/2(Out2) -> Out2/1  "Module Case Temp"
  In1/1 -> Inverter Thermal Model/1(In1)  "Pack Voltage"
  Inverter Thermal Model/3(Out3) -> Out3/1  "Coolant out Temp"
  Inverter Thermal Model/1(Out1) -> Out1/1  "Electrical Device Temps"
  In3/1 -> Coolant Properties/1(T_cool [K]), Inverter Thermal Model/3(In3)  "Coolant Temp, in"
  In2/1 -> Inverter Thermal Model/2(In2)  "RMS_Current"

== system Powertrain_Simulation/Motorcycle Model/Powertrain/Powertrain Thermal Model/EMRAX Motor Thermal Model/3-Mass Motor Thermal Model ==
  "Mass 1 : Stator Block" : Subsystem
  Mass 2 :Rotor Block : Subsystem
  "Mass 3 : Motor Mounting" : Subsystem
  T1 [K] : Outport
  T_cool_out [K] : Outport  Port=2
  T2 [K] : Outport  Port=3
  T3 [K] : Outport  Port=4
  wires:
  [Q_dot] -> Mass 2 :Rotor Block/1(Q_dot_heat [W]), "Mass 1 : Stator Block"/1(Q_dot_heat [W])
  Mass 2 :Rotor Block/1(T2 [K]) -> "Mass 3 : Motor Mounting"/1("T2 "), "Mass 1 : Stator Block"/2(T2 [K]), T2 [K]/1
  [T_cool_in] -> "Mass 1 : Stator Block"/3(T_cool_in [K])
  "Mass 1 : Stator Block"/1(T1 [K]) -> Mass 2 :Rotor Block/2(T1), T1 [K]/1
  [m_dot_cool] -> "Mass 1 : Stator Block"/4(m_dot_cool [kg/s])
  "Mass 1 : Stator Block"/2(T_cool_out) -> T_cool_out [K]/1
  "Mass 3 : Motor Mounting"/1(T3 [K]) -> Mass 2 :Rotor Block/3(T3), T3 [K]/1

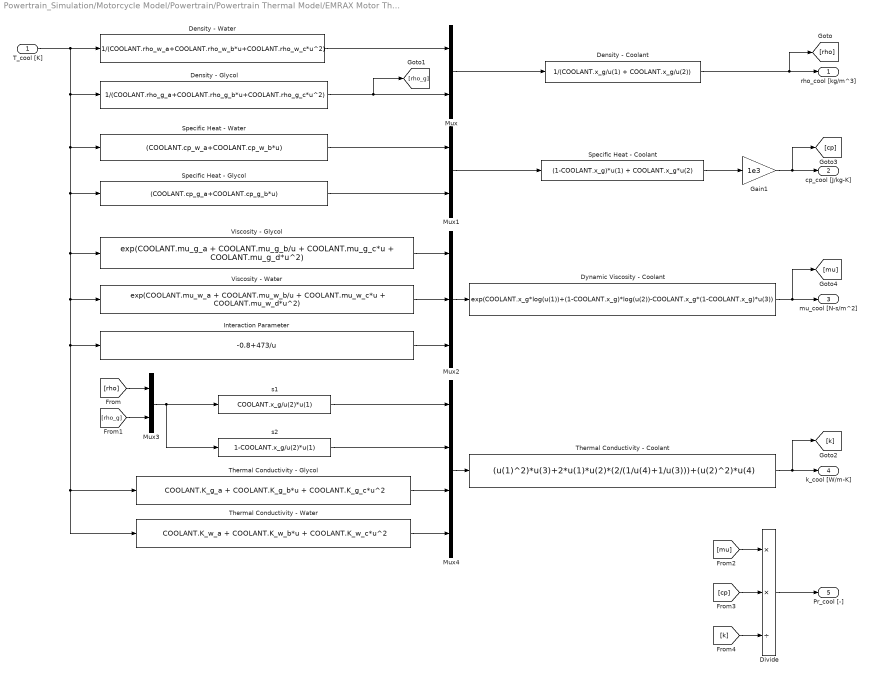
== system Powertrain_Simulation/Motorcycle Model/Powertrain/Powertrain Thermal Model/EMRAX Motor Thermal Model/Coolant Properties ==
  T_cool [K] : Inport
  Density - Coolant : Fcn  Expr=1/(COOLANT.x_g/u(1) + COOLANT.x_g/u(2))
  Density - Glycol : Fcn  Expr=1/(COOLANT.rho_g_a+COOLANT.rho_g_b*u+COOLANT.rho_g_c*u^2)
  Density - Water : Fcn  Expr=1/(COOLANT.rho_w_a+COOLANT.rho_w_b*u+COOLANT.rho_w_c*u^2)
  Divide : Product  Inputs=**/
  Dynamic Viscosity - Coolant : Fcn  Expr=exp(COOLANT.x_g*log(u(1))+(1-COOLANT.x_g)*log(u(2))-COOLANT.x_g*(1-COOLANT.x_g)*u(3))
  Gain1 : Gain  Gain=1e3
  Interaction Parameter : Fcn  Expr=-0.8+473/u
  Mux : Mux  Inputs=2
  Mux1 : Mux  Inputs=2
  Mux2 : Mux  Inputs=3
  Mux3 : Mux  Inputs=2
  Mux4 : Mux
  Specific Heat - Coolant : Fcn  Expr=(1-COOLANT.x_g)*u(1) + COOLANT.x_g*u(2)
  Specific Heat - Glycol : Fcn  Expr=(COOLANT.cp_g_a+COOLANT.cp_g_b*u)
  Specific Heat - Water : Fcn  Expr=(COOLANT.cp_w_a+COOLANT.cp_w_b*u)
  Thermal Conductivity - Coolant : Fcn  Expr=(u(1)^2)*u(3)+2*u(1)*u(2)*(2/(1/u(4)+1/u(3)))+(u(2)^2)*u(4)
  Thermal Conductivity - Glycol : Fcn  Expr=COOLANT.K_g_a + COOLANT.K_g_b*u + COOLANT.K_g_c*u^2
  Thermal Conductivity - Water : Fcn  Expr=COOLANT.K_w_a + COOLANT.K_w_b*u + COOLANT.K_w_c*u^2
  Viscosity - Glycol : Fcn  Expr=exp(COOLANT.mu_g_a + COOLANT.mu_g_b/u + COOLANT.mu_g_c*u + COOLANT.mu_g_d*u^2)
  Viscosity - Water : Fcn  Expr=exp(COOLANT.mu_w_a + COOLANT.mu_w_b/u + COOLANT.mu_w_c*u + COOLANT.mu_w_d*u^2)
  s1 : Fcn  Expr=COOLANT.x_g/u(2)*u(1)
  s2 : Fcn  Expr=1-COOLANT.x_g/u(2)*u(1)
  rho_cool [kg/m^3] : Outport
  cp_cool [J/kg-K] : Outport  Port=2
  mu_cool [N-s/m^2] : Outport  Port=3
  k_cool [W/m-K] : Outport  Port=4
  Pr_cool [-] : Outport  Port=5
  wires:
  Density - Coolant/1 -> rho_cool [kg/m^3]/1, [rho]
  Mux/1 -> Density - Coolant/1
  T_cool [K]/1 -> Density - Water/1, Density - Glycol/1, Specific Heat - Water/1, Specific Heat - Glycol/1, Viscosity - Glycol/1, Viscosity - Water/1, Interaction Parameter/1, Thermal Conductivity - Glycol/1, Thermal Conductivity - Water/1
  Specific Heat - Coolant/1 -> Gain1/1
  Gain1/1 -> cp_cool [J/kg-K]/1, [cp]
  Mux2/1 -> Dynamic Viscosity - Coolant/1
  Viscosity - Glycol/1 -> Mux2/1
  Viscosity - Water/1 -> Mux2/2
  Interaction Parameter/1 -> Mux2/3
  Density - Water/1 -> Mux/1
  Density - Glycol/1 -> Mux/2, [rho_g]
  Dynamic Viscosity - Coolant/1 -> mu_cool [N-s/m^2]/1, [mu]
  Specific Heat - Water/1 -> Mux1/1
  Specific Heat - Glycol/1 -> Mux1/2
  Mux1/1 -> Specific Heat - Coolant/1
  Thermal Conductivity - Glycol/1 -> Mux4/3
  Thermal Conductivity - Water/1 -> Mux4/4
  Mux4/1 -> Thermal Conductivity - Coolant/1
  [rho] -> Mux3/1
  [rho_g] -> Mux3/2
  Mux3/1 -> s1/1, s2/1
  s1/1 -> Mux4/1
  s2/1 -> Mux4/2
  Thermal Conductivity - Coolant/1 -> k_cool [W/m-K]/1, [k]
  Divide/1 -> Pr_cool [-]/1
  [mu] -> Divide/1
  [cp] -> Divide/2
  [k] -> Divide/3

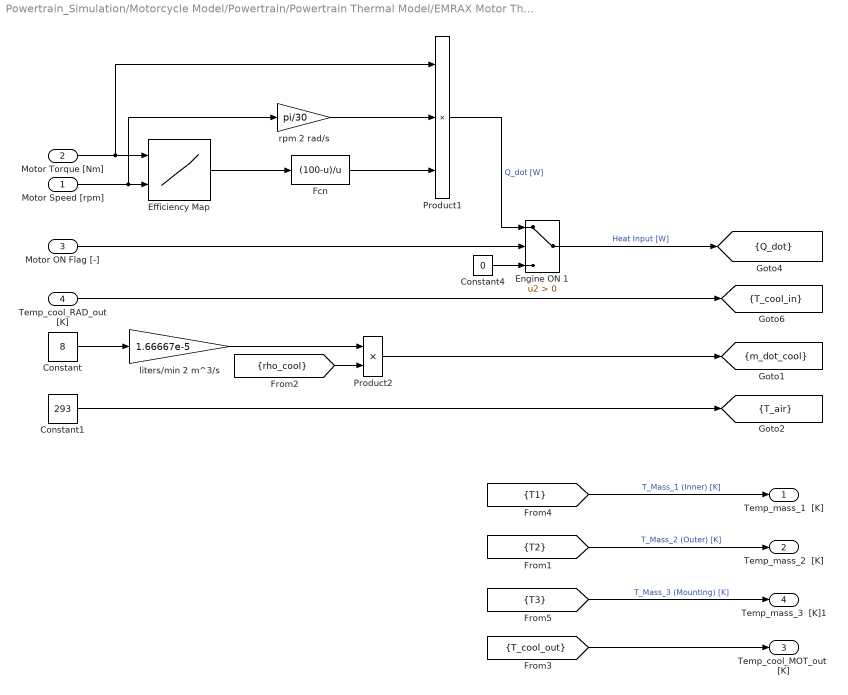
== system Powertrain_Simulation/Motorcycle Model/Powertrain/Powertrain Thermal Model/EMRAX Motor Thermal Model/Parameter Definition ==
  Motor Speed [rpm] : Inport
  Motor Torque [Nm] : Inport  Port=2
  Motor ON Flag [-] : Inport  Port=3
  Temp_cool_RAD_out [K] : Inport  Port=4
  Constant : Constant  Value=8
  Constant1 : Constant  Value=293
  Constant4 : Constant  Value=0
  Efficiency Map : Lookup_n-D  BreakpointsForDimension1=MOT.RPM  BreakpointsForDimension2=MOT.Torque  Table=MOT.eta'  ExtrapMethod=Clip  UseLastTableValue=on  RndMeth=Simplest  InputSameDT=on
  Engine ON 1 : Switch  Criteria=u2 > Threshold
  Fcn : Fcn  Expr=(100-u)/u
  Product1 : Product  Inputs=3
  Product2 : Product
  liters/min 2 m^3/s : Gain  Gain=1.66667e-5
  rpm 2 rad/s : Gain  Gain=pi/30
  Temp_mass_1  [K] : Outport
  Temp_mass_2  [K] : Outport  Port=2
  Temp_cool_MOT_out  [K] : Outport  Port=3
  Temp_mass_3  [K]1 : Outport  Port=4
  tag scope: Q_dot=scoped, T_air=scoped, T_cool_in=scoped, m_dot_cool=scoped
  wires:
  [T1] -> Temp_mass_1  [K]/1  "T_Mass_1 (Inner) [K]"
  [T2] -> Temp_mass_2  [K]/1  "T_Mass_2 (Outer) [K]"
  Temp_cool_RAD_out [K]/1 -> [T_cool_in]
  Constant4/1 -> Engine ON 1/3
  Engine ON 1/1 -> [Q_dot]  "Heat Input [W]"
  Motor ON Flag [-]/1 -> Engine ON 1/2
  Motor Torque [Nm]/1 -> Product1/1, Efficiency Map/1
  Motor Speed [rpm]/1 -> rpm 2 rad/s/1, Efficiency Map/2
  Constant/1 -> liters/min 2 m^3/s/1
  Efficiency Map/1 -> Fcn/1
  rpm 2 rad/s/1 -> Product1/2
  Fcn/1 -> Product1/3
  Product1/1 -> Engine ON 1/1  "Q_dot [W]"
  liters/min 2 m^3/s/1 -> Product2/1
  [rho_cool] -> Product2/2
  Product2/1 -> [m_dot_cool]
  Constant1/1 -> [T_air]
  [T_cool_out] -> Temp_cool_MOT_out  [K]/1
  [T3] -> Temp_mass_3  [K]1/1  "T_Mass_3 (Mounting) [K]"

== system Powertrain_Simulation/Motorcycle Model/Powertrain/Powertrain Thermal Model/Radiator Thermal Model/Air Properties ==
  T_air_in [K] : Inport
  Constant1 : Constant  Value=353.08
  Divide2 : Product  Inputs=*/
  Specific Heat - Air : Fcn  Expr=(AIR.cpair_a + AIR.cpair_b*u + AIR.cpair_c*u^2 + AIR.cpair_d*u^3 + AIR.cpair_e*u^4)*287
  rho_air [kg/m^3] : Outport
  cp_air [J/kg-K] : Outport  Port=2
  wires:
  Constant1/1 -> Divide2/1
  T_air_in [K]/1 -> Specific Heat - Air/1, Divide2/2
  Specific Heat - Air/1 -> cp_air [J/kg-K]/1  "cpair"
  Divide2/1 -> rho_air [kg/m^3]/1

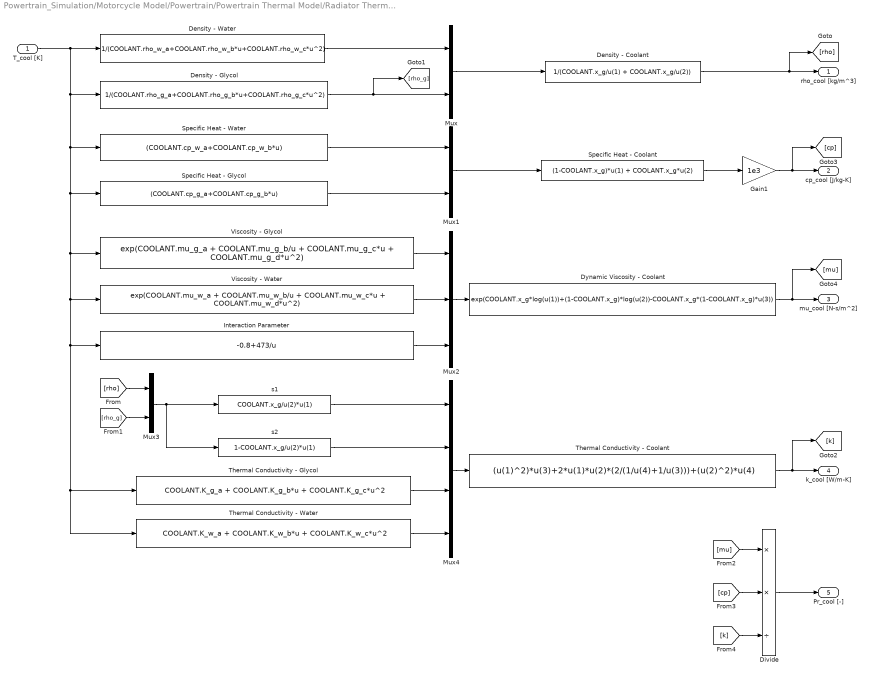
== system Powertrain_Simulation/Motorcycle Model/Powertrain/Powertrain Thermal Model/Radiator Thermal Model/Coolant Properties ==
  T_cool [K] : Inport
  Density - Coolant : Fcn  Expr=1/(COOLANT.x_g/u(1) + COOLANT.x_g/u(2))
  Density - Glycol : Fcn  Expr=1/(COOLANT.rho_g_a+COOLANT.rho_g_b*u+COOLANT.rho_g_c*u^2)
  Density - Water : Fcn  Expr=1/(COOLANT.rho_w_a+COOLANT.rho_w_b*u+COOLANT.rho_w_c*u^2)
  Divide : Product  Inputs=**/
  Dynamic Viscosity - Coolant : Fcn  Expr=exp(COOLANT.x_g*log(u(1))+(1-COOLANT.x_g)*log(u(2))-COOLANT.x_g*(1-COOLANT.x_g)*u(3))
  Gain1 : Gain  Gain=1e3
  Interaction Parameter : Fcn  Expr=-0.8+473/u
  Mux : Mux  Inputs=2
  Mux1 : Mux  Inputs=2
  Mux2 : Mux  Inputs=3
  Mux3 : Mux  Inputs=2
  Mux4 : Mux
  Specific Heat - Coolant : Fcn  Expr=(1-COOLANT.x_g)*u(1) + COOLANT.x_g*u(2)
  Specific Heat - Glycol : Fcn  Expr=(COOLANT.cp_g_a+COOLANT.cp_g_b*u)
  Specific Heat - Water : Fcn  Expr=(COOLANT.cp_w_a+COOLANT.cp_w_b*u)
  Thermal Conductivity - Coolant : Fcn  Expr=(u(1)^2)*u(3)+2*u(1)*u(2)*(2/(1/u(4)+1/u(3)))+(u(2)^2)*u(4)
  Thermal Conductivity - Glycol : Fcn  Expr=COOLANT.K_g_a + COOLANT.K_g_b*u + COOLANT.K_g_c*u^2
  Thermal Conductivity - Water : Fcn  Expr=COOLANT.K_w_a + COOLANT.K_w_b*u + COOLANT.K_w_c*u^2
  Viscosity - Glycol : Fcn  Expr=exp(COOLANT.mu_g_a + COOLANT.mu_g_b/u + COOLANT.mu_g_c*u + COOLANT.mu_g_d*u^2)
  Viscosity - Water : Fcn  Expr=exp(COOLANT.mu_w_a + COOLANT.mu_w_b/u + COOLANT.mu_w_c*u + COOLANT.mu_w_d*u^2)
  s1 : Fcn  Expr=COOLANT.x_g/u(2)*u(1)
  s2 : Fcn  Expr=1-COOLANT.x_g/u(2)*u(1)
  rho_cool [kg/m^3] : Outport
  cp_cool [J/kg-K] : Outport  Port=2
  mu_cool [N-s/m^2] : Outport  Port=3
  k_cool [W/m-K] : Outport  Port=4
  Pr_cool [-] : Outport  Port=5
  wires:
  Density - Coolant/1 -> rho_cool [kg/m^3]/1, [rho]
  Mux/1 -> Density - Coolant/1
  T_cool [K]/1 -> Density - Water/1, Density - Glycol/1, Specific Heat - Water/1, Specific Heat - Glycol/1, Viscosity - Glycol/1, Viscosity - Water/1, Interaction Parameter/1, Thermal Conductivity - Glycol/1, Thermal Conductivity - Water/1
  Specific Heat - Coolant/1 -> Gain1/1
  Gain1/1 -> cp_cool [J/kg-K]/1, [cp]
  Mux2/1 -> Dynamic Viscosity - Coolant/1
  Viscosity - Glycol/1 -> Mux2/1
  Viscosity - Water/1 -> Mux2/2
  Interaction Parameter/1 -> Mux2/3
  Density - Water/1 -> Mux/1
  Density - Glycol/1 -> Mux/2, [rho_g]
  Dynamic Viscosity - Coolant/1 -> mu_cool [N-s/m^2]/1, [mu]
  Specific Heat - Water/1 -> Mux1/1
  Specific Heat - Glycol/1 -> Mux1/2
  Mux1/1 -> Specific Heat - Coolant/1
  Thermal Conductivity - Glycol/1 -> Mux4/3
  Thermal Conductivity - Water/1 -> Mux4/4
  Mux4/1 -> Thermal Conductivity - Coolant/1
  [rho] -> Mux3/1
  [rho_g] -> Mux3/2
  Mux3/1 -> s1/1, s2/1
  s1/1 -> Mux4/1
  s2/1 -> Mux4/2
  Thermal Conductivity - Coolant/1 -> k_cool [W/m-K]/1, [k]
  Divide/1 -> Pr_cool [-]/1
  [mu] -> Divide/1
  [cp] -> Divide/2
  [k] -> Divide/3

== system Powertrain_Simulation/Motorcycle Model/Powertrain/Powertrain Thermal Model/Radiator Thermal Model/Reduced Radiator Thermal Model (1 Node - 1 Mass) ==
  T_cool_in [K] : Inport
  q_cool_in [m^3/s] : Inport  Port=2
  T_air [K] : Inport  Port=3
  V_face [m/s] : Inport  Port=4
  Divide3 : Product  Inputs=****
  Node 1 : Subsystem
  Sum3 : Sum  Inputs=+-
  T_cool_out [K] : Outport
  Q_dot_RAD [W] : Outport  Port=2
  wires:
  T_cool_in [K]/1 -> Node 1/1(T_c_in), Sum3/1
  T_air [K]/1 -> Node 1/3(T_air)
  Node 1/1(Tc) -> Sum3/2, T_cool_out [K]/1
  Sum3/1 -> Divide3/4
  [rho_cool] -> Divide3/1
  [cp_cool] -> Divide3/2
  Divide3/1 -> Q_dot_RAD [W]/1
  V_face [m/s]/1 -> Node 1/4(Vf)
  q_cool_in [m^3/s]/1 -> Divide3/3, Node 1/2(q_c)

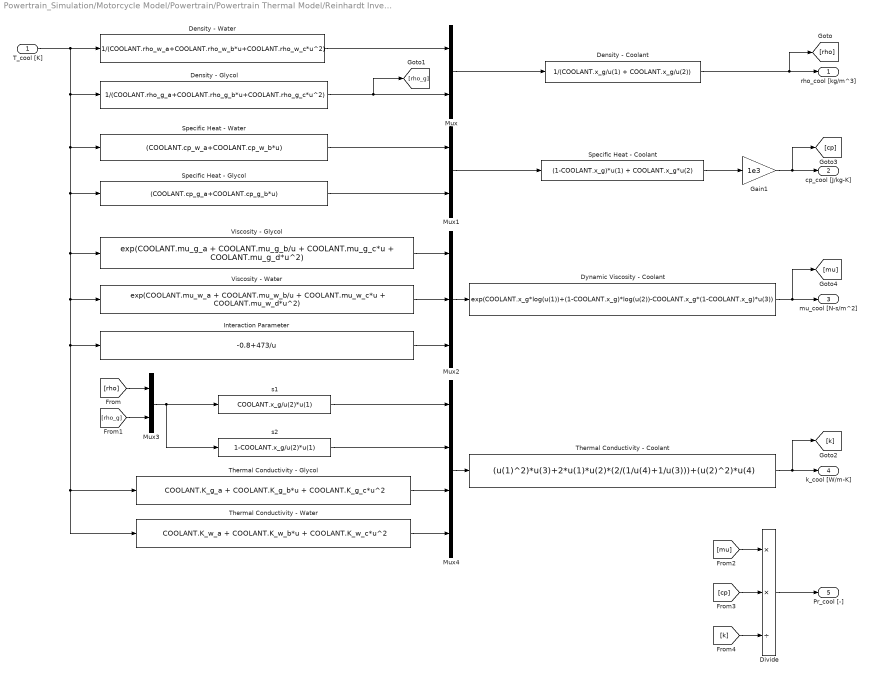
== system Powertrain_Simulation/Motorcycle Model/Powertrain/Powertrain Thermal Model/Reinhardt Inverter Thermal Model/Coolant Properties ==
  T_cool [K] : Inport
  Density - Coolant : Fcn  Expr=1/(COOLANT.x_g/u(1) + COOLANT.x_g/u(2))
  Density - Glycol : Fcn  Expr=1/(COOLANT.rho_g_a+COOLANT.rho_g_b*u+COOLANT.rho_g_c*u^2)
  Density - Water : Fcn  Expr=1/(COOLANT.rho_w_a+COOLANT.rho_w_b*u+COOLANT.rho_w_c*u^2)
  Divide : Product  Inputs=**/
  Dynamic Viscosity - Coolant : Fcn  Expr=exp(COOLANT.x_g*log(u(1))+(1-COOLANT.x_g)*log(u(2))-COOLANT.x_g*(1-COOLANT.x_g)*u(3))
  Gain1 : Gain  Gain=1e3
  Interaction Parameter : Fcn  Expr=-0.8+473/u
  Mux : Mux  Inputs=2
  Mux1 : Mux  Inputs=2
  Mux2 : Mux  Inputs=3
  Mux3 : Mux  Inputs=2
  Mux4 : Mux
  Specific Heat - Coolant : Fcn  Expr=(1-COOLANT.x_g)*u(1) + COOLANT.x_g*u(2)
  Specific Heat - Glycol : Fcn  Expr=(COOLANT.cp_g_a+COOLANT.cp_g_b*u)
  Specific Heat - Water : Fcn  Expr=(COOLANT.cp_w_a+COOLANT.cp_w_b*u)
  Thermal Conductivity - Coolant : Fcn  Expr=(u(1)^2)*u(3)+2*u(1)*u(2)*(2/(1/u(4)+1/u(3)))+(u(2)^2)*u(4)
  Thermal Conductivity - Glycol : Fcn  Expr=COOLANT.K_g_a + COOLANT.K_g_b*u + COOLANT.K_g_c*u^2
  Thermal Conductivity - Water : Fcn  Expr=COOLANT.K_w_a + COOLANT.K_w_b*u + COOLANT.K_w_c*u^2
  Viscosity - Glycol : Fcn  Expr=exp(COOLANT.mu_g_a + COOLANT.mu_g_b/u + COOLANT.mu_g_c*u + COOLANT.mu_g_d*u^2)
  Viscosity - Water : Fcn  Expr=exp(COOLANT.mu_w_a + COOLANT.mu_w_b/u + COOLANT.mu_w_c*u + COOLANT.mu_w_d*u^2)
  s1 : Fcn  Expr=COOLANT.x_g/u(2)*u(1)
  s2 : Fcn  Expr=1-COOLANT.x_g/u(2)*u(1)
  rho_cool [kg/m^3] : Outport
  cp_cool [J/kg-K] : Outport  Port=2
  mu_cool [N-s/m^2] : Outport  Port=3
  k_cool [W/m-K] : Outport  Port=4
  Pr_cool [-] : Outport  Port=5
  wires:
  Density - Coolant/1 -> rho_cool [kg/m^3]/1, [rho]
  Mux/1 -> Density - Coolant/1
  T_cool [K]/1 -> Density - Water/1, Density - Glycol/1, Specific Heat - Water/1, Specific Heat - Glycol/1, Viscosity - Glycol/1, Viscosity - Water/1, Interaction Parameter/1, Thermal Conductivity - Glycol/1, Thermal Conductivity - Water/1
  Specific Heat - Coolant/1 -> Gain1/1
  Gain1/1 -> cp_cool [J/kg-K]/1, [cp]
  Mux2/1 -> Dynamic Viscosity - Coolant/1
  Viscosity - Glycol/1 -> Mux2/1
  Viscosity - Water/1 -> Mux2/2
  Interaction Parameter/1 -> Mux2/3
  Density - Water/1 -> Mux/1
  Density - Glycol/1 -> Mux/2, [rho_g]
  Dynamic Viscosity - Coolant/1 -> mu_cool [N-s/m^2]/1, [mu]
  Specific Heat - Water/1 -> Mux1/1
  Specific Heat - Glycol/1 -> Mux1/2
  Mux1/1 -> Specific Heat - Coolant/1
  Thermal Conductivity - Glycol/1 -> Mux4/3
  Thermal Conductivity - Water/1 -> Mux4/4
  Mux4/1 -> Thermal Conductivity - Coolant/1
  [rho] -> Mux3/1
  [rho_g] -> Mux3/2
  Mux3/1 -> s1/1, s2/1
  s1/1 -> Mux4/1
  s2/1 -> Mux4/2
  Thermal Conductivity - Coolant/1 -> k_cool [W/m-K]/1, [k]
  Divide/1 -> Pr_cool [-]/1
  [mu] -> Divide/1
  [cp] -> Divide/2
  [k] -> Divide/3

== system Powertrain_Simulation/Motorcycle Model/Powertrain/Powertrain Thermal Model/Reinhardt Inverter Thermal Model/Inverter Thermal Model ==
  In1 : Inport
  In2 : Inport  Port=2
  In3 : Inport  Port=3
  Coolant Temp : Subsystem
  Heat Loss Calc (q_dot) : Fcn  Expr=0.000244*u(1)^1.072*u(2)^1.695+456.4
  Inverter Electrical Devices : Subsystem
  Module Case Temp : Subsystem
  Mux : Mux  Inputs=2
  Out1 : Outport
  Out2 : Outport  Port=2
  Out3 : Outport  Port=3
  tag scope: T_cool_in=global
  wires:
  In1/1 -> Mux/1  "Pack Voltage"
  In2/1 -> Mux/2  "RMS_Current"
  Mux/1 -> Heat Loss Calc (q_dot)/1
  Heat Loss Calc (q_dot)/1 -> Inverter Electrical Devices/1(Heat Rejection)
  Inverter Electrical Devices/1(Electrical Device Temps) -> Out1/1, Inverter Electrical Devices/2(Module Case Temp), Module Case Temp/1(Heat Rejection)  "Electrical Device Temps"
  Module Case Temp/1(Electrical Device Temps) -> Out2/1, Coolant Temp/1(Module Case Temp), Module Case Temp/2(Module Case Temp), Inverter Electrical Devices/3(In1)  "Module Case Temp"
  In3/1 -> [T_cool_in], Coolant Temp/2(Module Case Temp1), Module Case Temp/3(Module Case Temp1)  "Coolant Temp, in"
  Coolant Temp/1(Electrical Device Temps) -> Out3/1  "Coolant Temp, out"

== system Powertrain_Simulation/Motorcycle Model/Powertrain/Powertrain Thermal Model/EMRAX Motor Thermal Model/3-Mass Motor Thermal Model/Mass 1 : Stator Block ==
  note: Energy Balance for Mass 1 (Inner Mass)
  Q_dot_heat [W] : Inport
  T2 [K] : Inport  Port=2
  T_cool_in [K] : Inport  Port=3
  m_dot_cool [kg/s] : Inport  Port=4
  Gain : Gain  Gain=1/(MOT.M1*MOT.C1)
  Gain1 : Gain  Gain=MOT.alpha
  Gain2 : Gain  Gain=MOT.UA1
  Gain5 : Gain  Gain=MOT.k12
  Integrator : Integrator  InitialCondition=MOT.T_init
  Product1 : Product  Inputs=*//
  Sum1 : Sum  Inputs=+-
  Sum2 : Sum  Inputs=+-
  Sum3 : Sum  Inputs=+--
  Sum5 : Sum
  T1 [K] : Outport
  T_cool_out : Outport  Port=2
  wires:
  Sum1/1 -> Gain5/1
  T2 [K]/1 -> Sum1/2
  Integrator/1 -> Sum1/1, Sum2/1, T1 [K]/1
  Sum3/1 -> Gain/1
  Q_dot_heat [W]/1 -> Gain1/1  "Engine Heat Rejection (W)"
  Gain/1 -> Integrator/1
  Gain1/1 -> Sum3/1
  Gain5/1 -> Sum3/2
  T_cool_in [K]/1 -> Sum5/1, Sum2/2
  Gain2/1 -> Product1/1, Sum3/3
  Sum2/1 -> Gain2/1
  [cp_cool] -> Product1/2
  m_dot_cool [kg/s]/1 -> Product1/3
  Product1/1 -> Sum5/2
  Sum5/1 -> T_cool_out/1

== system Powertrain_Simulation/Motorcycle Model/Powertrain/Powertrain Thermal Model/EMRAX Motor Thermal Model/3-Mass Motor Thermal Model/Mass 2 :Rotor Block ==
  note: Energy Balance for Mass 2 (Rotor Mass)
  Q_dot_heat [W] : Inport
  T1 : Inport  Port=2
  T3 : Inport  Port=3
  Gain : Gain  Gain=1/(MOT.M2*MOT.C2)
  Gain1 : Gain  Gain=1-MOT.alpha
  Gain2 : Gain  Gain=MOT.UA2
  Gain3 : Gain  Gain=MOT.k23
  Gain5 : Gain  Gain=MOT.k12
  Integrator : Integrator  InitialCondition=MOT.T_init
  Sum1 : Sum  Inputs=+-
  Sum2 : Sum  Inputs=+-
  Sum3 : Sum  Inputs=++--
  Sum4 : Sum  Inputs=+-
  T2 [K] : Outport
  wires:
  Gain1/1 -> Sum3/1
  Gain/1 -> Integrator/1
  Q_dot_heat [W]/1 -> Gain1/1  "Engine Heat Rejection (W)"
  Sum3/1 -> Gain/1
  Integrator/1 -> Sum4/1, Sum1/2, Sum2/1, T2 [K]/1
  Sum1/1 -> Gain5/1
  Gain5/1 -> Sum3/2
  T1/1 -> Sum1/1
  Gain2/1 -> Sum3/3
  Sum2/1 -> Gain2/1
  [T_air] -> Sum2/2
  Sum4/1 -> Gain3/1
  T3/1 -> Sum4/2
  Gain3/1 -> Sum3/4

== system Powertrain_Simulation/Motorcycle Model/Powertrain/Powertrain Thermal Model/EMRAX Motor Thermal Model/3-Mass Motor Thermal Model/Mass 3 : Motor Mounting ==
  note: Energy Balance for Mass 2 (Outer Mass)
  "T2 " : Inport
  Gain : Gain  Gain=1/(MOT.M3*MOT.C3)
  Gain2 : Gain  Gain=MOT.UA3
  Gain5 : Gain  Gain=MOT.k23
  Integrator : Integrator  InitialCondition=MOT.T_init
  Sum1 : Sum  Inputs=+-
  Sum2 : Sum  Inputs=+-
  Sum3 : Sum  Inputs=+-
  T3 [K] : Outport
  wires:
  Gain/1 -> Integrator/1
  Sum3/1 -> Gain/1
  Integrator/1 -> T3 [K]/1, Sum1/2, Sum2/1
  Sum1/1 -> Gain5/1
  "T2 "/1 -> Sum1/1
  Gain2/1 -> Sum3/2
  Sum2/1 -> Gain2/1
  [T_air] -> Sum2/2
  Gain5/1 -> Sum3/1

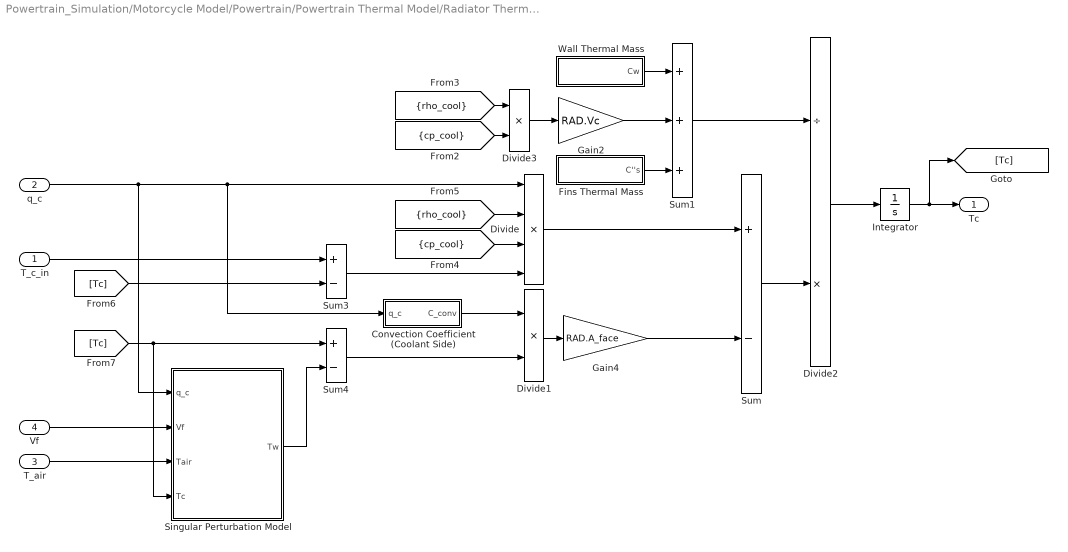
== system Powertrain_Simulation/Motorcycle Model/Powertrain/Powertrain Thermal Model/Radiator Thermal Model/Reduced Radiator Thermal Model (1 Node - 1 Mass)/Node 1 ==
  T_c_in : Inport
  q_c : Inport  Port=2
  T_air : Inport  Port=3
  Vf : Inport  Port=4
  Convection Coefficient (Coolant Side) : Subsystem
  Divide : Product  Inputs=****
  Divide1 : Product  Inputs=**
  Divide2 : Product  Inputs=/*
  Divide3 : Product  Inputs=**
  Fins Thermal Mass : Subsystem
  Gain2 : Gain  Gain=RAD.Vc
  Gain4 : Gain  Gain=RAD.A_face
  Integrator : Integrator  InitialCondition=RAD.T_init
  Singular Perturbation Model : Subsystem
  Sum : Sum  Inputs=+-
  Sum1 : Sum  Inputs=+++
  Sum3 : Sum  Inputs=+-
  Sum4 : Sum  Inputs=+-
  Wall Thermal Mass : Subsystem
  Tc : Outport
  wires:
  Convection Coefficient (Coolant Side)/1(C_conv) -> Divide1/1
  Gain2/1 -> Sum1/2
  Wall Thermal Mass/1(Cw) -> Sum1/1
  Fins Thermal Mass/1(C''s) -> Sum1/3
  Sum1/1 -> Divide2/1
  Integrator/1 -> Tc/1, [Tc]
  [rho_cool] -> Divide3/1
  [cp_cool] -> Divide3/2
  Divide3/1 -> Gain2/1
  Divide2/1 -> Integrator/1
  Sum/1 -> Divide2/2
  q_c/1 -> Convection Coefficient (Coolant Side)/1(q_c), Divide/1, Singular Perturbation Model/1(q_c)
  [rho_cool] -> Divide/2
  [cp_cool] -> Divide/3
  Divide/1 -> Sum/1
  Sum3/1 -> Divide/4
  T_c_in/1 -> Sum3/1
  [Tc] -> Sum3/2
  Gain4/1 -> Sum/2
  Divide1/1 -> Gain4/1
  Vf/1 -> Singular Perturbation Model/2(Vf)
  Sum4/1 -> Divide1/2
  [Tc] -> Singular Perturbation Model/4(Tc), Sum4/1
  T_air/1 -> Singular Perturbation Model/3(Tair)
  Singular Perturbation Model/1(Tw) -> Sum4/2
